simulink model "Interfaz"  (R2016a)
settings: Solver=VariableStepAuto  StartTime=0.0  StopTime=inf  RelTol=1e-3
values from neighbouring files (symbols this model uses):
  Asmc = [0 1;0 -Kf/I]    [Observador_Ivan.m]
  Bsmc = [0;Conv1*Kv*L1/I]    [Observador_Ivan.m]
  Csmc = [1 0]    [Observador_Ivan.m]
  Lsmc = PObs*Lbarra    [Observador_Ivan.m]
undefined symbols (not defined in the file or in its folder): K1
libraries: arduino_io_lib x5
settings Model: Creator=i95sa  LastModifiedBy=i95sa

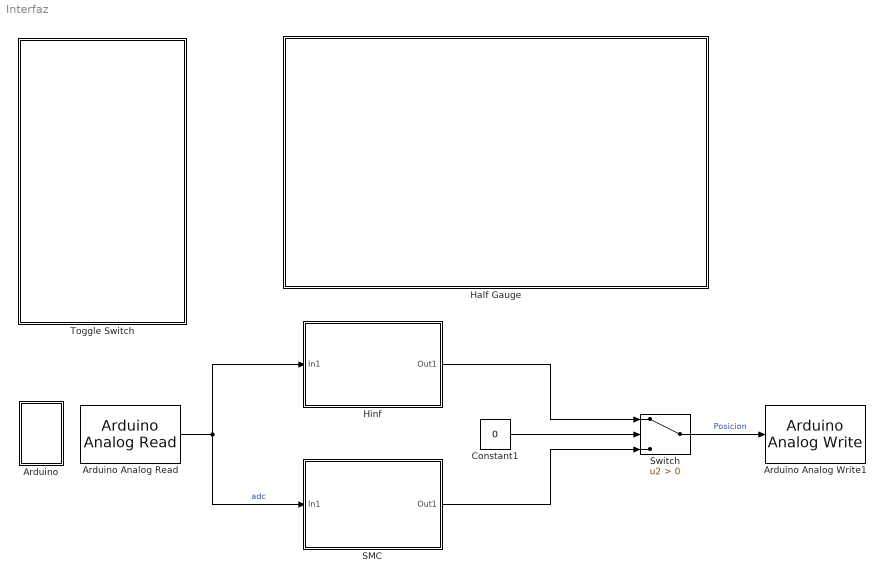
== system Interfaz ==
  Arduino : Subsystem
  Arduino Analog Read : arduino_io_lib/Arduino Analog Read  arduinoVar=Existing workspace arduino variable #1  arduinoPin=8  T=0.1
  Arduino Analog Write1 : arduino_io_lib/Arduino Analog Write  arduinoVar=Existing workspace arduino variable #1  arduinoPin=3  T=0.1
  Constant1 : Constant  Value=0
  Half Gauge : Subsystem  DialogController=hmiCreateDDGDialog  IsWebBlock=on  mask(MWDashboardBlock){webBlockId=320bc715-49a6-4852-8c54-a3e0fa69747f, webBlockType=semicirculargauge, ShowInLibBrowser=on, ShowInitialText=on, HMISrcModelName=Interfaz}
      mask prompts: webBlockId "WebBlock Id"; webBlockType "WebBlock Type"; HMISrcModelName "Source Model"
      mask Help: helpview([docroot '/mapfiles/simulink.map'], 'hmi_half_gauge')
      mask Display:
      | if strcmp(get_param(bdroot(gcb),'BlockDiagramType'), 'library')
      |     image([(matlabroot) '/toolbox/simulink/hmi/icons/SemicircularGauge.png']);
      | end
  Hinf : Subsystem
  SMC : Subsystem
  Switch : Switch  Criteria=u2 > Threshold
  Toggle Switch : Subsystem  DialogController=hmiCreateDDGDialog  IsWebBlock=on  mask(MWDashboardBlock){webBlockId=ecbc641e-6414-4af6-9af2-076ca0a8fad7, webBlockType=toggleswitch, ShowInLibBrowser=on, ShowInitialText=on, HMISrcModelName=Interfaz}
      mask prompts: webBlockId "WebBlock Id"; webBlockType "WebBlock Type"; HMISrcModelName "Source Model"
      mask Help: helpview([docroot '/mapfiles/simulink.map'], 'hmi_toggle_switch')
      mask Display:
      | if strcmp(get_param(bdroot(gcb),'BlockDiagramType'), 'library')
      |     image([(matlabroot) '/toolbox/simulink/hmi/icons/ToggleSwitch.png']);
      | end
  wires:
  Arduino Analog Read/1 -> Hinf/1(In1), SMC/1(In1)  "adc"
  Hinf/1(Out1) -> Switch/1
  SMC/1(Out1) -> Switch/3
  Switch/1 -> Arduino Analog Write1/1  "Posicion"
  Constant1/1 -> Switch/2

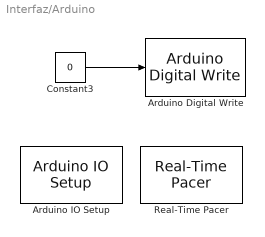
== system Interfaz/Arduino ==
  Arduino Digital Write : arduino_io_lib/Arduino Digital Write  arduinoVar=Existing workspace arduino variable #1  arduinoPin=12  T=0.1
  Arduino IO Setup : arduino_io_lib/Arduino IO Setup  Priority=3  arduinoVar=Existing workspace arduino variable #1  workspaceVarName=ard  comPort=4
  Constant3 : Constant  Value=0
  Real-Time Pacer : arduino_io_lib/Real-Time Pacer  simTimePerRealTime=1
  wires:
  Constant3/1 -> Arduino Digital Write/1

== system Interfaz/Half Gauge ==

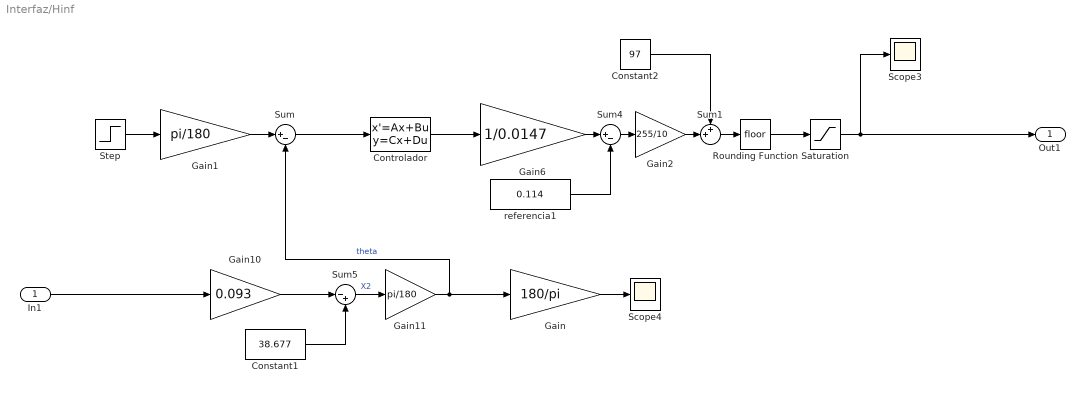
== system Interfaz/Hinf ==
  In1 : Inport
  Constant1 : Constant  Value=38.677
  Constant2 : Constant  Value=97
  Controlador : StateSpace  A=K1.a  B=K1.b  C=K1.c  D=K1.d  X0=0
  Gain : Gain  Gain=180/pi
  Gain1 : Gain  Gain=pi/180
  Gain10 : Gain  Gain=0.093
  Gain11 : Gain  Gain=pi/180
  Gain2 : Gain  Gain=255/10
  Gain6 : Gain  Gain=1/0.0147
  Rounding Function : Rounding
  Saturation : Saturate  UpperLimit=255  LowerLimit=0
  Scope3 : Scope
  Scope4 : Scope
  Step : Step  Time=0  After=0  SampleTime=0
  Sum : Sum  Inputs=|+-
  Sum1 : Sum  Inputs=++|
  Sum4 : Sum  Inputs=|+-
  Sum5 : Sum  Inputs=|-+
  referencia1 : Constant  Value=0.114
  Out1 : Outport
  wires:
  Controlador/1 -> Gain6/1
  Sum/1 -> Controlador/1
  Saturation/1 -> Out1/1, Scope3/1
  Constant2/1 -> Sum1/1
  Sum5/1 -> Gain11/1  "X2"
  In1/1 -> Gain10/1
  Sum4/1 -> Gain2/1
  Sum1/1 -> Rounding Function/1
  Constant1/1 -> Sum5/2
  Gain11/1 -> Gain/1, Sum/2  "theta"
  referencia1/1 -> Sum4/2
  Gain6/1 -> Sum4/1
  Gain1/1 -> Sum/1
  Rounding Function/1 -> Saturation/1
  Step/1 -> Gain1/1
  Gain/1 -> Scope4/1
  Gain2/1 -> Sum1/2
  Gain10/1 -> Sum5/1

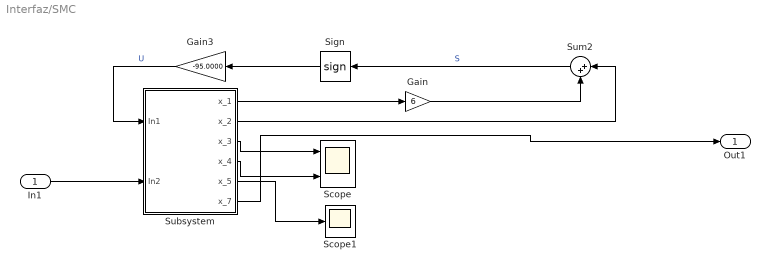
== system Interfaz/SMC ==
  In1 : Inport
  Gain : Gain  Gain=6
  Gain3 : Gain  Gain=-95.0000
  Scope : Scope  NumInputPorts=2
  Scope1 : Scope
  Sign : Signum  ZeroCross=off
  Subsystem : Subsystem
  Sum2 : Sum  Inputs=|++
  Out1 : Outport
  wires:
  Subsystem/4(x_4) -> Scope/2
  Subsystem/5(x_5) -> Scope1/1
  Gain3/1 -> Subsystem/1(In1)  "U"
  Sign/1 -> Gain3/1
  Sum2/1 -> Sign/1  "S"
  Subsystem/3(x_3) -> Scope/1
  Gain/1 -> Sum2/2
  Subsystem/1(x_1) -> Gain/1
  Subsystem/2(x_2) -> Sum2/1
  In1/1 -> Subsystem/2(In2)
  Subsystem/6(x_7) -> Out1/1

== system Interfaz/Toggle Switch ==

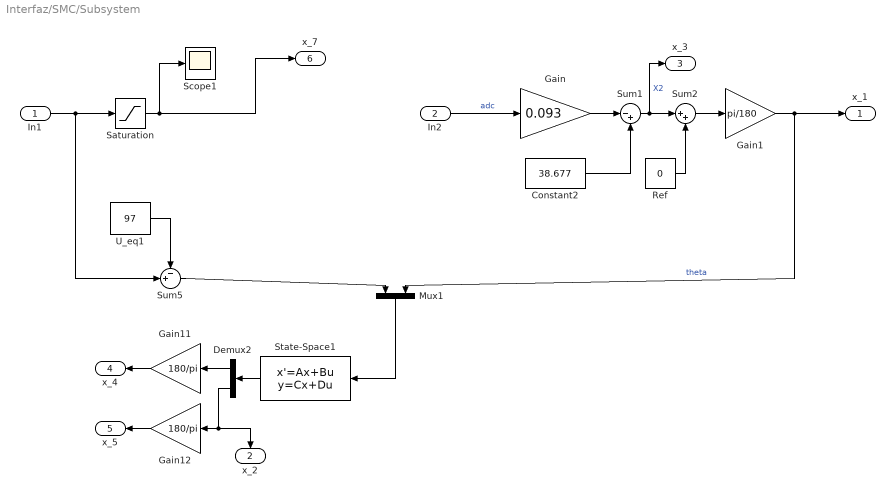
== system Interfaz/SMC/Subsystem ==
  In1 : Inport
  In2 : Inport  Port=2
  Constant2 : Constant  Value=38.677
  Demux2 : Demux  Outputs=2
  Gain : Gain  Gain=0.093
  Gain1 : Gain  Gain=pi/180
  Gain11 : Gain  Gain=180/pi
  Gain12 : Gain  Gain=180/pi
  Mux1 : Mux  Inputs=2
  Ref : Constant  Value=0
  Saturation : Saturate  UpperLimit=255  LowerLimit=80  ZeroCross=off
  Scope1 : Scope
  State-Space1 : StateSpace  A=Asmc-Lsmc*Csmc  B=[Bsmc Lsmc]  C=eye(2)  D=zeros(2,2)  X0=[-0.65 0]
  Sum1 : Sum  Inputs=|-+
  Sum2 : Sum  Inputs=|++
  Sum5 : Sum  Inputs=-+|
  U_eq1 : Constant  Value=97
  x_1 : Outport
  x_2 : Outport  Port=2
  x_3 : Outport  Port=3
  x_4 : Outport  Port=4
  x_5 : Outport  Port=5
  x_7 : Outport  Port=6
  wires:
  In2/1 -> Gain/1  "adc"
  Gain/1 -> Sum1/1
  Constant2/1 -> Sum1/2
  Gain1/1 -> x_1/1, Mux1/2  "theta"
  State-Space1/1 -> Demux2/1
  Mux1/1 -> State-Space1/1
  Sum5/1 -> Mux1/1
  U_eq1/1 -> Sum5/1
  Gain12/1 -> x_5/1
  Demux2/2 -> x_2/1, Gain12/1
  Demux2/1 -> Gain11/1
  Gain11/1 -> x_4/1
  In1/1 -> Sum5/2, Saturation/1
  Sum1/1 -> x_3/1, Sum2/1  "X2"
  Ref/1 -> Sum2/2
  Sum2/1 -> Gain1/1
  Saturation/1 -> x_7/1, Scope1/1
